simulink subsystem "pendulum"  (R2023b)
settings: Solver=VariableStepAuto  StartTime=0.0  StopTime=10.0  RelTol=1e-3
values from neighbouring files (symbols this model uses):
  g = 9.81    [linearized_sys.m]    (also in system_configuration.m)
  Kd = 10    [linearized_sys.m]    (also in system_configuration.m)
  L = 0.5    [linearized_sys.m]    (also in system_configuration.m)
  m = size(B1,2)    [constr_matrix.m]    (also in linearized_sys.m = 1; mpc_without_constr.m; system_configuration.m = 1)
  M = 1    [linearized_sys.m]    (also in system_configuration.m)
settings Model: Creator=aniello  LastModifiedBy=aniello

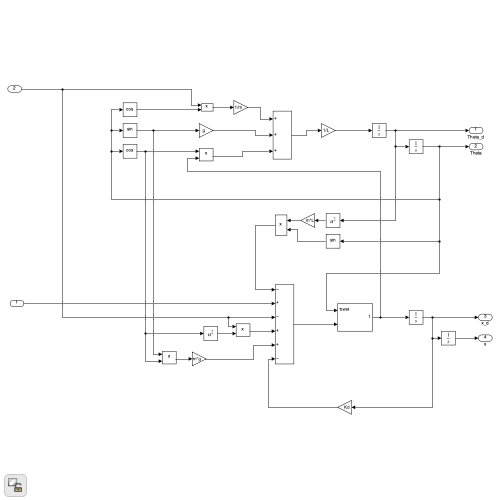
[thumbnail: Simulink's stored preview of the top-level diagram]
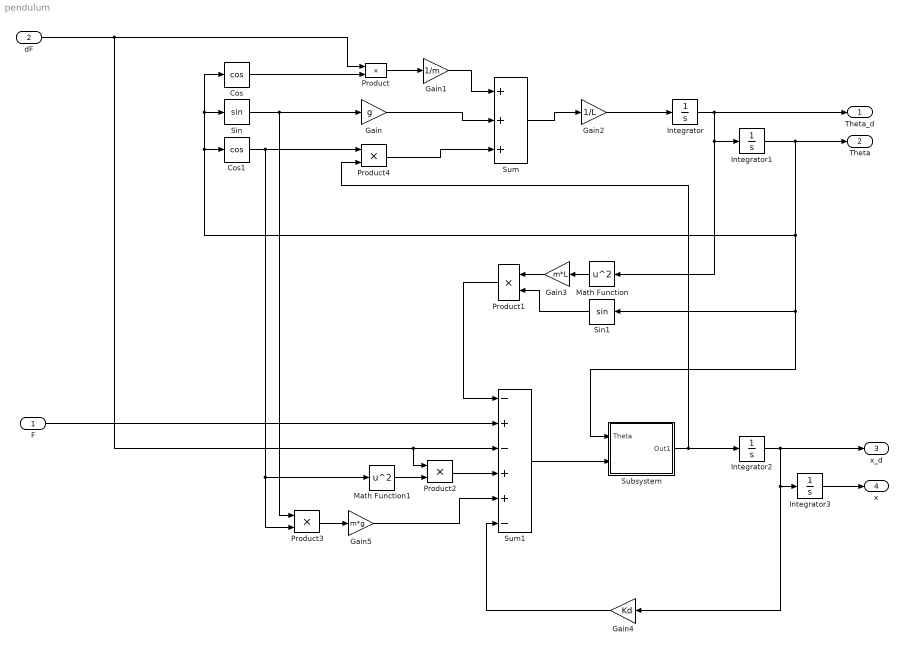
== system pendulum ==
  F : Inport
  dF : Inport  Port=2
  Cos : Trigonometry  Operator=cos
  Cos1 : Trigonometry  Operator=cos
  Gain : Gain  Gain=g
  Gain1 : Gain  Gain=1/m
  Gain2 : Gain  Gain=1/L
  Gain3 : Gain  Gain=m*L
  Gain4 : Gain  Gain=Kd
  Gain5 : Gain  Gain=m*g
  Integrator{,1..3} (4 alike) : Integrator
  Math Function : Math  Operator=square
  Math Function1 : Math  Operator=square
  Product{,1..4} (5 alike) : Product
  Sin : Trigonometry
  Sin1 : Trigonometry
  Subsystem : Subsystem
  Sum : Sum  Inputs=+++
  Sum1 : Sum  Inputs=-+-++-
  Theta_d : Outport
  Theta : Outport  Port=2  Unit=rad/s
  x_d : Outport  Port=3
  x : Outport  Port=4  Unit=m
  wires:
  Cos/1 -> Product/2
  Gain/1 -> Sum/2
  dF/1 -> Product2/1, Sum1/3, Product/1
  Sum/1 -> Gain2/1
  Gain1/1 -> Sum/1
  Gain4/1 -> Sum1/6
  Subsystem/1(Out1) -> Product4/2, Integrator2/1
  Gain5/1 -> Sum1/5
  Sin1/1 -> Product1/2
  Integrator2/1 -> x_d/1, Integrator3/1, Gain4/1
  Product1/1 -> Sum1/1
  Integrator1/1 -> Theta/1, Cos1/1, Cos/1, Sin/1, Sin1/1, Subsystem/1(Theta)
  Product/1 -> Gain1/1
  F/1 -> Sum1/2
  Math Function/1 -> Gain3/1
  Product3/1 -> Gain5/1
  Product2/1 -> Sum1/4
  Sin/1 -> Gain/1, Product3/1
  Sum1/1 -> Subsystem/2(.)
  Gain2/1 -> Integrator/1
  Math Function1/1 -> Product2/2
  Cos1/1 -> Product3/2, Math Function1/1, Product4/1
  Gain3/1 -> Product1/1
  Integrator/1 -> Theta_d/1, Math Function/1, Integrator1/1
  Integrator3/1 -> x/1
  Product4/1 -> Sum/3

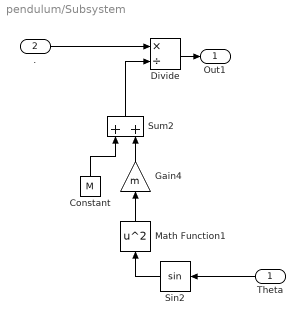
== system pendulum/Subsystem ==
  Theta : Inport
  . : Inport  Port=2
  Constant : Constant  Value=M
  Divide : Product  Inputs=*/
  Gain4 : Gain  Gain=m
  Math Function1 : Math  Operator=square
  Sin2 : Trigonometry
  Sum2 : Sum
  Out1 : Outport
  wires:
  ./1 -> Divide/1
  Sin2/1 -> Math Function1/1
  Theta/1 -> Sin2/1
  Constant/1 -> Sum2/1
  Sum2/1 -> Divide/2
  Math Function1/1 -> Gain4/1
  Divide/1 -> Out1/1
  Gain4/1 -> Sum2/2
